simulink model "Increment_and_Decrement_Timer_2018b"  (R2018b)
settings: Solver=FixedStepDiscrete  StartTime=0.0  StopTime=20  FixedStep=0.1  RelTol=1e-3
settings Model: Creator=eness  LastModifiedBy=eness
settings DataIOCC: ReturnWorkspaceOutputs=on
settings DebuggingCC: UnconnectedInputMsg=none  UnconnectedOutputMsg=none  UnconnectedLineMsg=none  SFMachineParentedDataDiag=error
settings ModelReferenceCC: EnableRefExpFcnMdlSchedulingChecks=off
settings RTWCC: Description=Generic Real-Time Target

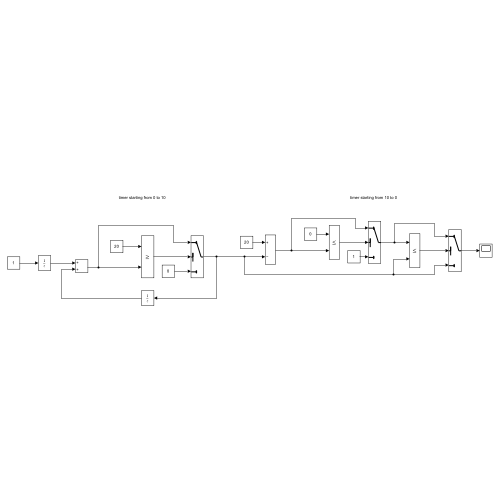
[thumbnail: Simulink's stored preview of the top-level diagram]
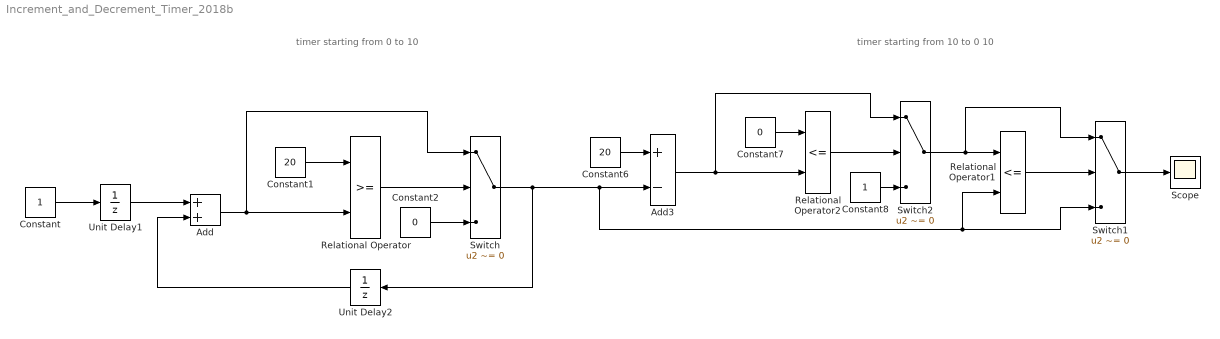
== system Increment_and_Decrement_Timer_2018b ==
  note: timer starting from 0 to 10
  note: timer starting from 10 to 0 10
  Add : Sum
  Add3 : Sum  Inputs=+-
  Constant : Constant
  Constant1 : Constant  Value=20
  Constant2 : Constant  Value=0
  Constant6 : Constant  Value=20
  Constant7 : Constant  Value=0
  Constant8 : Constant
  Relational Operator : RelationalOperator  OutDataTypeStr=boolean  RndMeth=Simplest
  Relational Operator1 : RelationalOperator  Operator=<=  OutDataTypeStr=boolean  RndMeth=Simplest
  Relational Operator2 : RelationalOperator  Operator=<=  OutDataTypeStr=boolean  RndMeth=Simplest
  Scope : Scope
  Switch : Switch  Criteria=u2 ~= 0
  Switch1 : Switch  Criteria=u2 ~= 0
  Switch2 : Switch  Criteria=u2 ~= 0
  Unit Delay1 : UnitDelay  SampleTime=-1  HasFrameUpgradeWarning=on
  Unit Delay2 : UnitDelay  SampleTime=-1  HasFrameUpgradeWarning=on
  wires:
  Constant1/1 -> Relational Operator/1
  Relational Operator/1 -> Switch/2
  Add/1 -> Relational Operator/2, Switch/1
  Unit Delay1/1 -> Add/1
  Constant/1 -> Unit Delay1/1
  Unit Delay2/1 -> Add/2
  Constant2/1 -> Switch/3
  Constant8/1 -> Switch2/3
  Constant7/1 -> Relational Operator2/1
  Relational Operator2/1 -> Switch2/2
  Constant6/1 -> Add3/1
  Add3/1 -> Switch2/1, Relational Operator2/2
  Switch/1 -> Unit Delay2/1, Switch1/3, Relational Operator1/2, Add3/2
  Switch2/1 -> Switch1/1, Relational Operator1/1
  Relational Operator1/1 -> Switch1/2
  Switch1/1 -> Scope/1
